simulink model "Exercise_2"  (R2020b)
settings: Solver=VariableStepAuto  StartTime=0.0  StopTime=0.01  RelTol=1e-3
libraries: fl_lib x10, nesl_utility x3, ee_lib x1
settings Model: Creator=zaliyazici  LastModifiedBy=zaliyazici

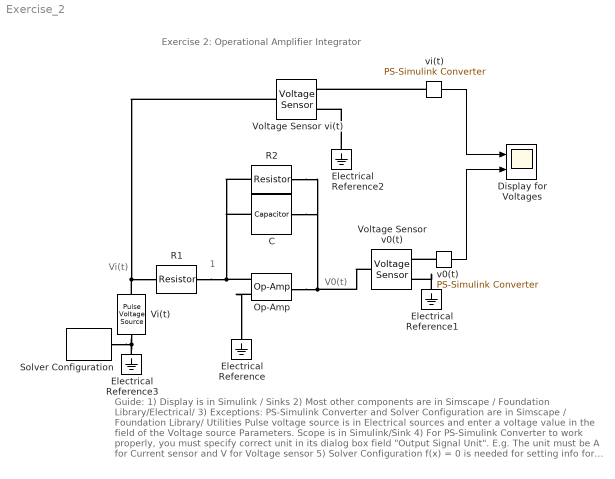
== system Exercise_2 ==
  note: V0(t)
  note: Guide:
      | 1) Display is in Simulink / Sinks
      | 2) Most other components are in Simscape / Foundation Library/Electrical/
      | 3) Exceptions: PS-Simulink Converter and Solver Configuration are in Simscape / Foundation Library/ Utilities
      | Pulse voltage source is in Electrical sources and enter a voltage value in the field of the Voltage source Parameters.
      | Scope is in Simulink/Sink
      | 4) For PS-Simulink Converter to work properly, you must specify correct unit in its dialog box field "Output Signal Unit".
      | E.g. The unit must be A for Current sensor and V for Voltage sensor
      | 5) Solver Configuration f(x) = 0 is needed for setting info for simulation.
      | 6) To create "Annotation", double-click a location on project page and select "Create annotation" from the prompt. Then, type any text you want to clarify your circuit. E.g. "Display for Voltage".
      | 7) To understand how to use a component, right-click on the component and select "Help".
      | Measurement: Node voltages $v_i(t)$ , and $v_0(t)$
  note: Exercise 2: Operational Amplifier Integrator
  note: 1
  note: Vi(t)
  C : fl_lib/Electrical/Electrical Elements/Capacitor  c=10 uF  r=1e-6 Ohm  g=0 1/Ohm  i_specify=off  i_priority=None  i=0 A  i_nominal_specify=off  i_nominal_unit=A  i_nominal_value=1  v_specify=off  v_priority=None  v=0 V  v_nominal_specify=off  v_nominal_unit=V  v_nominal_value=1  vc_specify=off  vc_priority=High  vc=0 V  vc_nominal_specify=off  vc_nominal_unit=V  vc_nominal_value=1
      settings: AttributesFormatString=%<c> %<c_unit>
  Display for Voltages : Scope  NumInputPorts=2
  Electrical Reference{,1..3} (4 alike) : fl_lib/Electrical/Electrical Elements/Electrical Reference
  "Op-Amp " : fl_lib/Electrical/Electrical Elements/Op-Amp  outI_specify=off  outI_priority=None  outI=0 A  outI_nominal_specify=off  outI_nominal_unit=A  outI_nominal_value=1
  R1 : fl_lib/Electrical/Electrical Elements/Resistor  R=1 kOhm  i_specify=off  i_priority=None  i=0 A  i_nominal_specify=off  i_nominal_unit=A  i_nominal_value=1  v_specify=off  v_priority=None  v=0 V  v_nominal_specify=off  v_nominal_unit=V  v_nominal_value=1
      settings: AttributesFormatString=%<R> %<R_unit>  LogSimulationData=on
  R2 : fl_lib/Electrical/Electrical Elements/Resistor  R=5 kOhm  i_specify=off  i_priority=None  i=0 A  i_nominal_specify=off  i_nominal_unit=A  i_nominal_value=1  v_specify=off  v_priority=None  v=0 V  v_nominal_specify=off  v_nominal_unit=V  v_nominal_value=1
      settings: AttributesFormatString=%<R> %<R_unit>  LogSimulationData=on
  Solver Configuration : nesl_utility/Solver Configuration  PhysicalDomain=network_engine_domain  SubClassName=solver  LeftPortType=input  RightPortType=generic  Tones=[]  Harmonics=[]  SimulateNoise=off  Profile=off  UseLocalSampling=off  EnableSwitchedLinearOptims=on  FrequencyDomain=off  UseCCode=off  RelTol=0.001  AbsTol=1e-06  MinStep=1e-09  ToWorkspace=off  RevertToSquareIcSolve=off  NumHomotopyIterations=100  PhasorMode=off  PhasorModeNumHarmonics=1  DoDC=off  ResidualTolerance=1e-09  UseLocalSolver=off  LocalSolverChoice=NE_BACKWARD_EULER_ADVANCER  LocalSolverSampleTime=0.001  DoFixedCost=off  MaxNonlinIter=3  MaxModeIter=2  ComputeImpulses=off  ImpulseIterations=2  LinearAlgebra=auto  EquationFormulation=NE_TIME_EF  DelaysMemoryBudget=1024  AutomaticFiltering=on  FilteringTimeConstant=0.001  PartitionStorageMethod=AS_NEEDED  PartitionMemoryBudget=1024  PartitionMethod=ROBUST
  Vi(t) : ee_lib/Additional Components/SPICE Sources/Pulse Voltage Source  V1=2 V  V2=-2 V  TD=0 s  TR=1e-9 ms  TF=1e-9 ms  PW=1-1e-9 ms  PER=2 ms
      settings: SourceProductBaseCode=PS  InternalSimscapePortConfiguration="{\"Bottom\":[],\"Left\":[{\"id\":\"p\",\"label\":\"\",\"type\":\"foundation.electrical.electrical\"}],\"Right\":[{\"id\":\"n\",\"label\":\"\",\"type\":\"foundation.electrical.electrical\"}],\"Top\":[]}"
  Voltage Sensor v0(t) : fl_lib/Electrical/Electrical Sensors/Voltage Sensor
  Voltage Sensor vi(t) : fl_lib/Electrical/Electrical Sensors/Voltage Sensor
  v0(t) : nesl_utility/PS-Simulink Converter  PhysicalDomain=network_engine_domain  SubClassName=ps_output  LeftPortType=input  RightPortType=output  PseudoPeriodic=off  Frequencies=[]  Unit=V  AffineConversion=off
  vi(t) : nesl_utility/PS-Simulink Converter  PhysicalDomain=network_engine_domain  SubClassName=ps_output  LeftPortType=input  RightPortType=output  PseudoPeriodic=off  Frequencies=[]  Unit=V  AffineConversion=off
  wires:
  v0(t)/1 -> Display for Voltages/2
  vi(t)/1 -> Display for Voltages/1
  connections:
  Vi(t)/LConn1 -- Voltage Sensor vi(t)/LConn1 -- R1/LConn1
  "Op-Amp "/LConn1 -- Electrical Reference/LConn1
  Electrical Reference1/LConn1 -- Voltage Sensor v0(t)/RConn2
  v0(t)/LConn1 -- Voltage Sensor v0(t)/RConn1
  vi(t)/LConn1 -- Voltage Sensor vi(t)/RConn1
  "Op-Amp "/RConn1 -- R2/LConn1 -- C/LConn1 -- Voltage Sensor v0(t)/LConn1
  Electrical Reference2/LConn1 -- Voltage Sensor vi(t)/RConn2
  Solver Configuration/RConn1 -- Vi(t)/RConn1 -- Electrical Reference3/LConn1
  R1/RConn1 -- R2/RConn1 -- C/RConn1 -- "Op-Amp "/LConn2
